simulink model "ADC_SPWM_Openloop_2"  (R2024b)
settings: Solver=FixedStepDiscrete  StartTime=0.0  StopTime=inf  FixedStep=Ts  RelTol=1e-3
model workspace (MAT data in the model file):
  f = 25
undefined symbols (not defined in the file): alpha, C28x, CPU1, CPU2, DiscIntNeverNeededParam, Down, dspblkCoreblockFVToolHelper, gcbh, GPTRIP1SEL, T_period, Ts, TZ1, Up
libraries: c2802xlib x22, c2837xDlib x2, dspstat3 x2, c280xlib x2, simulink x1, mcbpositiondecoderlib x1
(part 2 of 2)

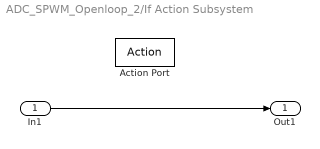
== system ADC_SPWM_Openloop_2/If Action Subsystem ==
  In1 : Inport
  Action Port : ActionPort  ActionPortLabel=if(u1 > 0.005)
  Out1 : Outport
  wires:
  In1/1 -> Out1/1

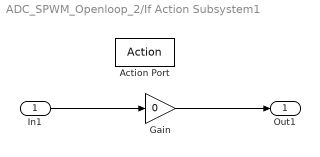
== system ADC_SPWM_Openloop_2/If Action Subsystem1 ==
  In1 : Inport
  Action Port : ActionPort  ActionPortLabel=else
  Gain : Gain  Gain=0
  Out1 : Outport
  wires:
  In1/1 -> Gain/1
  Gain/1 -> Out1/1

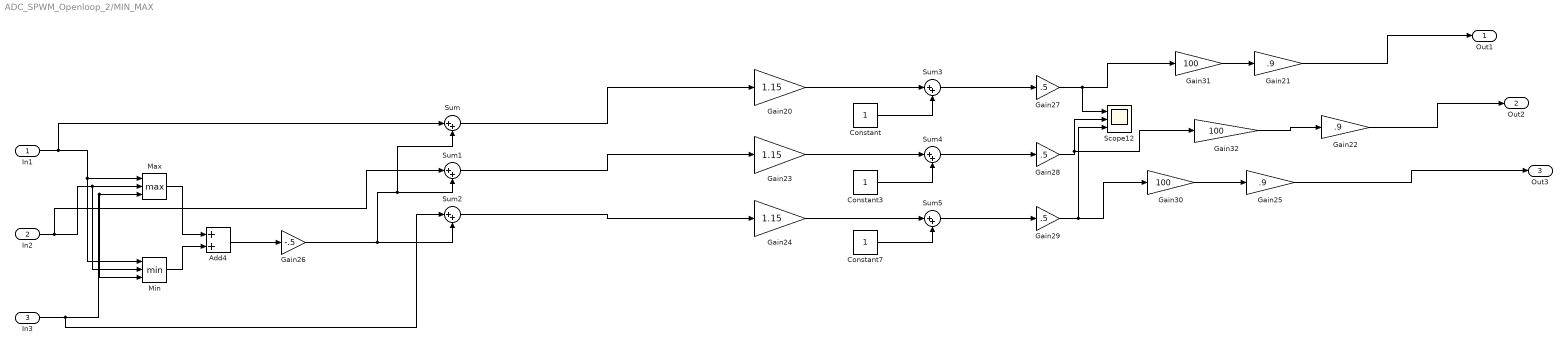
== system ADC_SPWM_Openloop_2/MIN_MAX ==
  In1 : Inport
  In2 : Inport  Port=2
  In3 : Inport  Port=3
  Add4 : Sum
  Constant : Constant
  Constant3 : Constant
  Constant7 : Constant
  Gain20 : Gain  Gain=1.15
  Gain21 : Gain  Gain=.9
  Gain22 : Gain  Gain=.9
  Gain23 : Gain  Gain=1.15
  Gain24 : Gain  Gain=1.15
  Gain25 : Gain  Gain=.9
  Gain26 : Gain  Gain=-.5
  Gain27 : Gain  Gain=.5
  Gain28 : Gain  Gain=.5
  Gain29 : Gain  Gain=.5
  Gain30 : Gain  Gain=100
  Gain31 : Gain  Gain=100
  Gain32 : Gain  Gain=100
  Max : MinMax  Function=max  Inputs=3
  Min : MinMax  Inputs=3
  Scope12 : Scope  NumInputPorts=3
  Sum{,1..5} (6 alike) : Sum  Inputs=|++
  Out1 : Outport
  Out2 : Outport  Port=2
  Out3 : Outport  Port=3
  wires:
  Gain28/1 -> Scope12/2, Gain32/1
  Sum3/1 -> Gain27/1
  In1/1 -> Sum/1, Min/1, Max/1
  Gain32/1 -> Gain22/1
  In3/1 -> Sum2/1, Min/3, Max/3
  Gain29/1 -> Scope12/3, Gain30/1
  In2/1 -> Sum1/1, Min/2, Max/2
  Constant7/1 -> Sum5/2
  Sum/1 -> Gain20/1
  Gain26/1 -> Sum/2, Sum1/2, Sum2/2
  Add4/1 -> Gain26/1
  Gain30/1 -> Gain25/1
  Min/1 -> Add4/2
  Gain20/1 -> Sum3/1
  Gain27/1 -> Scope12/1, Gain31/1
  Constant3/1 -> Sum4/2
  Gain24/1 -> Sum5/1
  Constant/1 -> Sum3/2
  Sum4/1 -> Gain28/1
  Gain21/1 -> Out1/1
  Sum1/1 -> Gain23/1
  Max/1 -> Add4/1
  Gain25/1 -> Out3/1
  Gain31/1 -> Gain21/1
  Sum2/1 -> Gain24/1
  Gain23/1 -> Sum4/1
  Sum5/1 -> Gain29/1
  Gain22/1 -> Out2/1

== matlab function ADC_SPWM_Openloop_2/MATLAB Function1 ==
  data: u input; y output; f input; Ts input; numPeriods input
function y = dcOffset_longWindow(u, f, Ts, numPeriods)
% u            : input signal (sine wave + offset)
% f            : frequency of the sine wave (Hz)
% Ts           : sample time (s)
% numPeriods   : number of periods to average over (e.g., 10)
% y            : output = DC offset (running average from first sample)

persistent buffer sumBuf idx N count

if isempty(N)
    samplesPerPeriod = round(1 / (f * Ts));
    N = samplesPerPeriod * numPeriods;   % total window length
    buffer = zeros(N, 1);
    sumBuf = 0;
    idx = 1;
    count = 0;          % number of samples received so far
end

% Update circular buffer: subtract oldest only if buffer is already full
if count >= N
    % Full window mode: subtract the sample that will be overwritten
    sumBuf = sumBuf - buffer(idx);
else
    % Startup mode: no subtraction, just accumulating
    % (buffer initially zeros, so subtracting would incorrectly remove zeros)
end

% Store new sample and update sum
buffer(idx) = u;
sumBuf = sumBuf + u;
idx = mod(idx, N) + 1;
count = count + 1;

% Output the average over the actual number of samples received so far
if count < N
    y = sumBuf / count;    % running average from first sample
else
    y = sumBuf / N;        % steady-state full‑window average
end
end

== matlab function ADC_SPWM_Openloop_2/MATLAB Function ==
  data: theta input; speed_rad_s output; Ts input
function speed_rad_s = calculate_speed(theta, Ts)
    % persistent variable remembers the angle from the previous time step
    persistent theta_prev;
    if isempty(theta_prev)
        theta_prev = 0;
    end

    % Calculate the raw delta
    delta_theta = theta - theta_prev;

    % UNWRAP LOGIC: Fix the jump from 2*pi to 0 (and vice versa)
    if delta_theta < -pi
        delta_theta = delta_theta + 2*pi;
    elseif delta_theta > pi
        delta_theta = delta_theta - 2*pi;
    end

    % Calculate speed and update previous value
    speed_rad_s = delta_theta / Ts;
    theta_prev = theta;
end

== matlab function ADC_SPWM_Openloop_2/MATLAB Function2 ==
  data: u input; y output; f input; Ts input; numPeriods input
function y = dcOffset_longWindow(u, f, Ts, numPeriods)
% u            : input signal (sine wave + offset)
% f            : frequency of the sine wave (Hz)
% Ts           : sample time (s)
% numPeriods   : number of periods to average over (e.g., 10)
% y            : output = DC offset (running average from first sample)

persistent buffer sumBuf idx N count

if isempty(N)
    samplesPerPeriod = round(1 / (f * Ts));
    N = samplesPerPeriod * numPeriods;   % total window length
    buffer = zeros(N, 1);
    sumBuf = 0;
    idx = 1;
    count = 0;          % number of samples received so far
end

% Update circular buffer: subtract oldest only if buffer is already full
if count >= N
    % Full window mode: subtract the sample that will be overwritten
    sumBuf = sumBuf - buffer(idx);
else
    % Startup mode: no subtraction, just accumulating
    % (buffer initially zeros, so subtracting would incorrectly remove zeros)
end

% Store new sample and update sum
buffer(idx) = u;
sumBuf = sumBuf + u;
idx = mod(idx, N) + 1;
count = count + 1;

% Output the average over the actual number of samples received so far
if count < N
    y = sumBuf / count;    % running average from first sample
else
    y = sumBuf / N;        % steady-state full‑window average
end
end

== matlab function ADC_SPWM_Openloop_2/MATLAB Function3 ==
  data: u input; y output; f input; Ts input; numPeriods input
function y = dcOffset_longWindow(u, f, Ts, numPeriods)
% u            : input signal (sine wave + offset)
% f            : frequency of the sine wave (Hz)
% Ts           : sample time (s)
% numPeriods   : number of periods to average over (e.g., 10)
% y            : output = DC offset (running average from first sample)

persistent buffer sumBuf idx N count

if isempty(N)
    samplesPerPeriod = round(1 / (f * Ts));
    N = samplesPerPeriod * numPeriods;   % total window length
    buffer = zeros(N, 1);
    sumBuf = 0;
    idx = 1;
    count = 0;          % number of samples received so far
end

% Update circular buffer: subtract oldest only if buffer is already full
if count >= N
    % Full window mode: subtract the sample that will be overwritten
    sumBuf = sumBuf - buffer(idx);
else
    % Startup mode: no subtraction, just accumulating
    % (buffer initially zeros, so subtracting would incorrectly remove zeros)
end

% Store new sample and update sum
buffer(idx) = u;
sumBuf = sumBuf + u;
idx = mod(idx, N) + 1;
count = count + 1;

% Output the average over the actual number of samples received so far
if count < N
    y = sumBuf / count;    % running average from first sample
else
    y = sumBuf / N;        % steady-state full‑window average
end
end

== matlab function ADC_SPWM_Openloop_2/MATLAB Function4 ==
  data: u input; y output; f input; Ts input; numPeriods input
function y = dcOffset_EMA(u, f, Ts, numPeriods)
%#codegen
% Exponential moving average - C-friendly
% Time constant = numPeriods * (1/f)

persistent alpha y_prev

if isempty(alpha)
    samplesPerPeriod = round(1 / (f * Ts));
    N = samplesPerPeriod * numPeriods;
    alpha = 1 / N;
    y_prev = u;
end

% First-order low-pass filter
y = y_prev + alpha * (u - y_prev);
y_prev = y;
end

== matlab function ADC_SPWM_Openloop_2/MATLAB Function5 ==
  data: u input; y output; f input; Ts input; numPeriods input
function y = dcOffset_EMA(u, f, Ts, numPeriods)
%#codegen
% Exponential moving average - C-friendly
% Time constant = numPeriods * (1/f)

persistent alpha y_prev

if isempty(alpha)
    samplesPerPeriod = round(1 / (f * Ts));
    N = samplesPerPeriod * numPeriods;
    alpha = 1 / N;
    y_prev = u;
end

% First-order low-pass filter
y = y_prev + alpha * (u - y_prev);
y_prev = y;
end

== matlab function ADC_SPWM_Openloop_2/MATLAB Function6 ==
  data: u input; y output; f input; Ts input; numPeriods input
function y = dcOffset_EMA(u, f, Ts, numPeriods)
%#codegen
% Exponential moving average - C-friendly
% Time constant = numPeriods * (1/f)

persistent alpha y_prev

if isempty(alpha)
    samplesPerPeriod = round(1 / (f * Ts));
    N = samplesPerPeriod * numPeriods;
    alpha = 1 / N;
    y_prev = u;
end

% First-order low-pass filter
y = y_prev + alpha * (u - y_prev);
y_prev = y;
end
